simulink model "dashboard2021b"  (R2022a)
settings: Solver=VariableStepAuto  StartTime=0.0  StopTime=inf  RelTol=1e-3
settings Model: Creator=bryantboatright  LastModifiedBy=bryantboatright
settings ModelReferenceCC: EnableRefExpFcnMdlSchedulingChecks=off
settings RTWCC: Description=Generic Real-Time Target

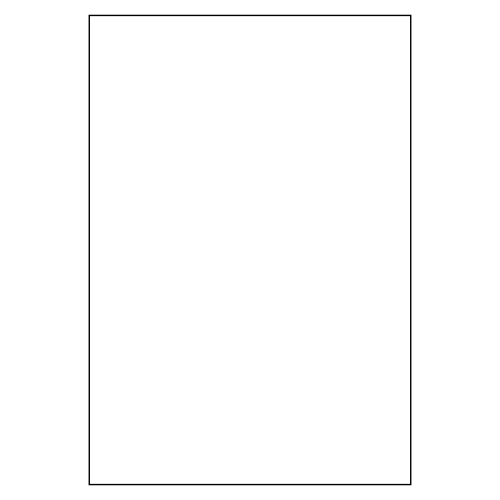
[thumbnail: Simulink's stored preview of the top-level diagram]
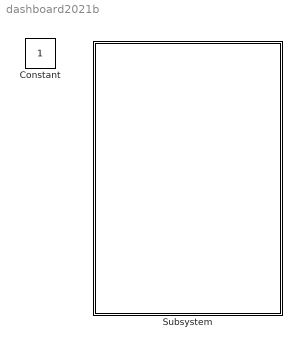
== system dashboard2021b ==
  Subsystem : Subsystem
  Constant : Constant  IOType=siggen

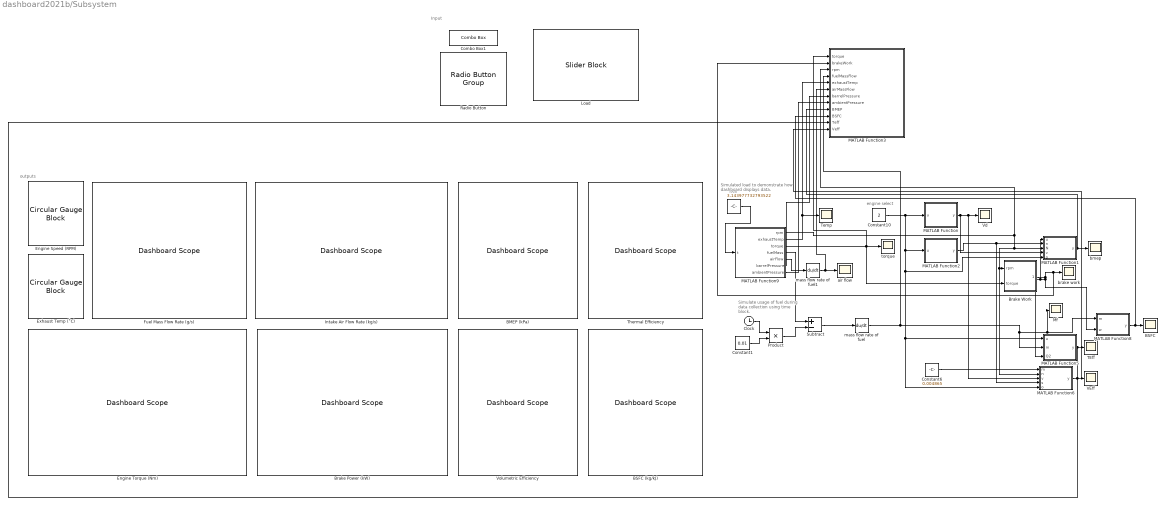
== system dashboard2021b/Subsystem ==
  note: Simulated load to demonstrate how
      | dashboard displays data.
  note: Simulate usage of fuel
      | during data collection
      | using time block.
  note: outputs
  note: Input
  note: engine select
  "\"load\"" : Constant  Value=3.143977732793522
  BMEP (kPa) : DashboardScope
  BSFC : Scope
  BSFC (kg/kJ) : DashboardScope
  Brake Power (kW) : DashboardScope
  Brake Work : MATLAB Function  TreatAsAtomicUnit=on
  Clock : Clock
  Combo Box1 : ComboBox  LabelPosition=Bottom  SelectedLabel=Craftsman
      settings: Values={{'Yanmar', 'Craftsman', 'John Deer', 'Chevy V6', 'Kohler', 'DuroMax'}, [1 2 3 4 5 6]}
  Constant1 : Constant  Value=0.01
  Constant10 : Constant  Value=2
  Constant6 : Constant  Value=0.004865
  Engine Speed (RPM) : CircularGaugeBlock  ScaleMax=7000
  Engine Torque (Nm) : DashboardScope
  Exhaust Temp (˚C) : CircularGaugeBlock  ScaleMax=1000
  Fuel Mass Flow Rate (g/s) : DashboardScope
  Intake Air Flow Rate (kg/s) : DashboardScope
  Load : SliderBlock
  MATLAB Function : MATLAB Function  TreatAsAtomicUnit=on
  MATLAB Function1 : MATLAB Function  TreatAsAtomicUnit=on
  MATLAB Function2 : MATLAB Function  TreatAsAtomicUnit=on
  MATLAB Function3 : MATLAB Function  TreatAsAtomicUnit=on  SystemSampleTime=1
  MATLAB Function5 : MATLAB Function  TreatAsAtomicUnit=on
  MATLAB Function6 : MATLAB Function  TreatAsAtomicUnit=on
  MATLAB Function8 : MATLAB Function  TreatAsAtomicUnit=on
  MATLAB Function9 : MATLAB Function  TreatAsAtomicUnit=on
  Mf : Scope
  Product : Product
  Radio Button : RadioButtonGroup  SelectedLabel=Metric  ButtonGroupName=Units
      settings: Values={{'Metric', 'Imperial'}, [0 1]}
  Subtract : Sum  Inputs=+-
  TEff : Scope
  Temp : Scope
  Thermal Efficiency : DashboardScope
  VEff : Scope
  Vd : Scope
  Volumetric Efficiency : DashboardScope
  air flow : Scope
  bmep : Scope
  brake work : Scope
  mass flow rate of fuel : Derivative
  mass flow rate of fuel1 : Derivative
  torque : Scope
  wires:
  Constant6/1 -> MATLAB Function6/1(m)
  MATLAB Function/1(y) -> MATLAB Function1/4(v), MATLAB Function6/3(v), Vd/1
  MATLAB Function2/1(y) -> MATLAB Function6/4(s), MATLAB Function1/2(n)
  MATLAB Function8/1(y) -> MATLAB Function3/10(BSFC), BSFC/1
  MATLAB Function1/1(y) -> MATLAB Function3/9(BMEP), bmep/1
  MATLAB Function6/1(y) -> MATLAB Function3/12(Veff), VEff/1
  Constant10/1 -> MATLAB Function1/5(o), MATLAB Function5/1(u), MATLAB Function6/5(o), MATLAB Function2/1(u), MATLAB Function/1(u)
  MATLAB Function5/1(y) -> MATLAB Function3/11(Teff), TEff/1
  Brake Work/1(brakeWork) -> MATLAB Function5/3(Q2), MATLAB Function1/1(u), MATLAB Function8/2(w), MATLAB Function3/2(brakeWork), brake work/1
  MATLAB Function9/1(rpm) -> MATLAB Function3/3(rpm), MATLAB Function6/2(n), Brake Work/1(rpm), MATLAB Function1/3(N)
  MATLAB Function9/2(exhaustTemp) -> MATLAB Function3/5(exhaustTemp), Temp/1
  MATLAB Function9/3(torque) -> Brake Work/2(torque), MATLAB Function3/1(torque), torque/1
  "\"load\""/1 -> MATLAB Function9/1(t)
  mass flow rate of fuel/1 -> MATLAB Function3/4(fuelMassFlow), MATLAB Function5/2(m), Mf/1, MATLAB Function8/1(m)
  MATLAB Function9/4(fuelMass) -> Subtract/1
  Subtract/1 -> mass flow rate of fuel/1
  Clock/1 -> Product/1
  Constant1/1 -> Product/2
  Product/1 -> Subtract/2
  mass flow rate of fuel1/1 -> MATLAB Function3/6(airMassFlow), air flow/1
  MATLAB Function9/5(airFlow) -> mass flow rate of fuel1/1
  MATLAB Function9/6(barrelPressure) -> MATLAB Function3/7(barrelPressure)
  MATLAB Function9/7(ambientPressure) -> MATLAB Function3/8(ambientPressure)

== matlab function dashboard2021b/Subsystem/MATLAB Function3 ==
  data: torque input; brakeWork input; rpm input; fuelMassFlow input; exhaustTemp input; airMassFlow input; barrelPressure input; ambientPressure input; BMEP input; BSFC input; Teff input; Veff input
% log file generation - currently overwrites each run
% \r\n used for windows line termination style CRLF - switch to just \n if
% using unix like system
function fileOutput(torque,brakeWork,rpm,fuelMassFlow,exhaustTemp,airMassFlow,barrelPressure,ambientPressure,BMEP,BSFC,Teff,Veff)

file = fopen('~/output-file.txt','w');
fprintf(file,'%.3f,%.3f,%.3f,%.3f,%.3f,%.3f,%.3f,%.3f,%.3f,%.3f,%.3f,%.3f\r\n', ...
torque,brakeWork,rpm,fuelMassFlow,exhaustTemp,airMassFlow,barrelPressure,ambientPressure,BMEP,BSFC,Teff,Veff);
fclose(file);

== matlab function dashboard2021b/Subsystem/MATLAB Function1 ==
  data: u input; y output; n input; N input; v input; o input
function y = fcn(u, n, N,  v, o)
if(o == 1 || o == 2 || o == 5 || o ==6)
    y = ((u/((N/60)/n))/v)/1000;
elseif(o==3)
     y = ((u/((N/60)/n))/(v*4))/1000;
else
     y = ((u/((N/60)/n))/(v*6))/1000;
end

== matlab function dashboard2021b/Subsystem/MATLAB Function ==
  data: y output; u input
function y = fcn(u)
data = [0.000296 0.000196 0.000475 000.0004667 0.000429 0.000225];

y = data(1,u);

== matlab function dashboard2021b/Subsystem/MATLAB Function2 ==
  data: y output; u input
function y = fcn(u)
data = [4  4  4  4 4 4];

y = data(1,u);

== matlab function dashboard2021b/Subsystem/Brake Work ==
  data: rpm input; brakeWork output; torque input
function brakeWork = fcn(rpm,torque)
brakeWork = 2 * pi * (rpm/60.0) * torque;

== matlab function dashboard2021b/Subsystem/MATLAB Function5 ==
  data: y output; u input; m input; Q2 input
function y = fcn(u, m, Q2)
data = [47.3e6 44.4e6];
Q1 = 0;
if(u == 3)
    Q1 = m * data(1, 2);

else
    Q1 = m * data(1,1);
end

y = (Q2/Q1) * 100;

== matlab function dashboard2021b/Subsystem/MATLAB Function6 ==
  data: m input; y output; n input; v input; s input; o input
function y = fcn(m, n, v, s,o)
if(o == 1 || o == 2 || o == 5 || o == 6)
    y = ((s*m)/(1.205*v*(n/60)));
elseif (o == 3)
    y = ((s*m)/(1.205*(v*4)*(n/60)));
else
    y = ((s*m)/(1.205*(v*6)*(n/60)));
end

== matlab function dashboard2021b/Subsystem/MATLAB Function8 ==
  data: m input; y output; w input
function y = fcn(m,w)

y = m./w;

== matlab function dashboard2021b/Subsystem/MATLAB Function9 ==
  data: rpm output; t input; exhaustTemp output; torque output; fuelMass output; airFlow output; barrelPressure output; ambientPressure output
% function to generate simulated engine values. Takes two values:
%   u: boolean on or off switch to start data collection.
%   t: float value to scale the simulated data, tied to a slider.
%
% returns:
%
%   rpm: engine     speed rev per minute
%   exhaustTemp:    exhaust temperature in celsius
%   torque:         torque in Newton-meters
%   torqueMeasured: boolean - true if torque is measured, false if not
%   volts:          voltage
%   amps:           current
%   fuelMass:       mass of fuel container at current time.

function [ rpm,exhaustTemp,torque,fuelMass,airFlow,barrelPressure,ambientPressure ] = fcn(t)
data = (1 + t / 100.0) * [ 2000 125 2.258 2.75 0.004 0.94 ];
rpm = data(1);
exhaustTemp = data(2);
torque = data(3);
fuelMass = data(4);
airFlow = data(5);
barrelPressure = data(6);
ambientPressure = 29;
